simulink model "inverseTest"  (R2018b)
settings: Solver=FixedStepDiscrete  StartTime=0.0  StopTime=100.0  FixedStep=0.2  RelTol=1e-3
values from neighbouring files (symbols this model uses):
  SS_discrete = c2d(SS_full,Ts)    [discreteInverse.m]
  SS_inverse = ss(SS_inverse.A, SS_inverse.B,SS_inverse.C,SS_inverse.D,-1)    [discreteInverse.m]
settings Model: Creator=user  LastModifiedBy=user

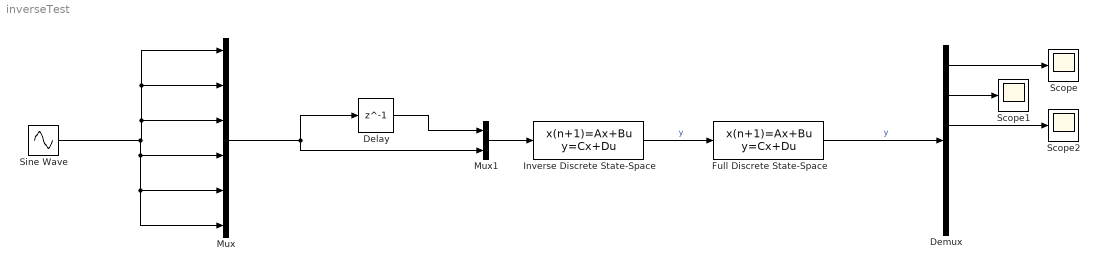
== system inverseTest ==
  Delay : Delay  DelayLength=1  InitialCondition=0
  Demux : Demux  Outputs=6
  Full Discrete State-Space : DiscreteStateSpace  A=SS_discrete.A  B=SS_discrete.B  C=SS_discrete.C  D=SS_discrete.D  SampleTime=-1
  Inverse Discrete State-Space : DiscreteStateSpace  A=SS_inverse.A  B=SS_inverse.B  C=SS_inverse.C  D=SS_inverse.D  SampleTime=-1
  Mux : Mux  Inputs=6
  Mux1 : Mux  Inputs=2
  Scope : Scope
  Scope1 : Scope
  Scope2 : Scope
  Sine Wave : Sin  Amplitude=1e6  Frequency=0.5  SampleTime=0
  wires:
  Full Discrete State-Space/1 -> Demux/1  "y"
  Sine Wave/1 -> Mux/6, Mux/5, Mux/4, Mux/3, Mux/2, Mux/1
  Demux/1 -> Scope/1
  Mux/1 -> Mux1/2, Delay/1
  Mux1/1 -> Inverse Discrete State-Space/1
  Inverse Discrete State-Space/1 -> Full Discrete State-Space/1  "y"
  Delay/1 -> Mux1/1
  Demux/2 -> Scope1/1
  Demux/3 -> Scope2/1
